simulink model "LQR_sim"  (R2018b)
settings: Solver=ode45  StartTime=0.0  StopTime=tf  RelTol=1e-3  EnableMultiTasking=on
values from neighbouring files (symbols this model uses):
  a = 0.92    [LQR.m]
  b = 0.5    [LQR.m]
  initial = [0,10]    [LQR.m]
  J = 6689.281*10^-6    (= 0.006689281)    [LQR.m]    (also in optimalcontrol.m)
  L = 284.84*10^-3    (= 0.28484)    [LQR.m]    (also in optimalcontrol.m = 0.5*R*u^2)
  PWMs_fixed = [1619,1638]    [LQR.m]
libraries: aerolibconvert2 x2
settings Model: Creator=lorem  LastModifiedBy=davidefontana
settings DataIOCC: LimitDataPoints=on  SaveFormat=Array
settings OptimizationCC: LifeSpan=inf
settings DebuggingCC: SolverPrmCheckMsg=warning  SFUnexpectedBacktrackingDiag=warning  SFNoUnconditionalDefaultTransitionDiag=warning  SFExecutionAtInitializationDiag=none
settings HardwareCC: ProdBitPerPointer=32  ProdBitPerSizeT=32  ProdBitPerPtrDiffT=32  ProdLargestAtomicFloat=None  ProdIntDivRoundTo=Undefined  ProdEndianess=Unspecified  ProdWordSize=32  ProdHWDeviceType=32-bit Generic
settings ModelReferenceCC: PropagateSignalLabelsOutOfModel=off
settings SFSimCC: SimUseLocalCustomCode=off
settings RTWCC: RTWUseLocalCustomCode=off
settings CodeAppCC: StateflowObjectComments=on
settings GRTTargetCC: TargetLangStandard=C89/C90 (ANSI)  GeneratePreprocessorConditionals=Disable all
settings ConfigComp: CovMetricSettings=dw  CovHtmlReporting=on  CovSaveCumulativeToWorkspaceVar=on  CovSaveSingleToWorkspaceVar=on  CovExternalEMLEnable=off  CovSFcnEnable=off

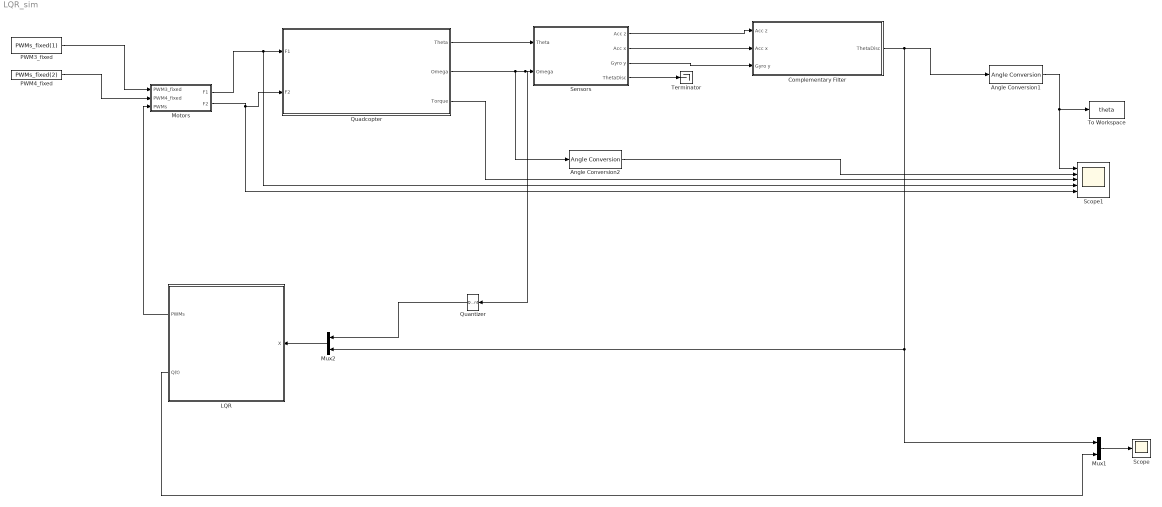
== system LQR_sim ==
  Angle Conversion1 : aerolibconvert2/Angle Conversion  IU=rad  OU=deg
  Angle Conversion2 : aerolibconvert2/Angle Conversion  IU=rad  OU=deg
  Complementary Filter : Subsystem
  LQR : Subsystem
  Motors : Subsystem
  Mux1 : Mux  Inputs=2
  Mux2 : Mux  Inputs=2
  PWM3_fixed : Constant  Value=PWMs_fixed(1)  SampleTime=0.02
  PWM4_fixed : Constant  Value=PWMs_fixed(2)  SampleTime=0.02
  Quadcopter : Subsystem
  Quantizer : Quantizer  QuantizationInterval=0.01  SampleTime=0.02
  Scope : Scope
  Scope1 : Scope  NumInputPorts=5
  Sensors : Subsystem
  Terminator : Terminator
  To Workspace : ToWorkspace  VariableName=theta  SaveFormat=Timeseries  SampleTime=-1
  wires:
  PWM4_fixed/1 -> Motors/2(PWM4_fixed)
  Motors/2(F2) -> Scope1/5, Quadcopter/2(F2)
  Motors/1(F1) -> Scope1/4, Quadcopter/1(F1)
  Sensors/3(Gyro y) -> Complementary Filter/3(Gyro y)
  Sensors/2(Acc x) -> Complementary Filter/2("Acc x ")
  Sensors/1(Acc z) -> Complementary Filter/1(Acc z)
  PWM3_fixed/1 -> Motors/1(PWM3_fixed)
  Angle Conversion1/1 -> Scope1/1, To Workspace/1
  Quadcopter/2(Omega) -> Quantizer/1, Sensors/2(Omega), Angle Conversion2/1
  Quadcopter/1(Theta) -> Sensors/1(Theta)
  Quadcopter/3("Torque ") -> Scope1/3
  Sensors/4(ThetaDisc) -> Terminator/1
  Angle Conversion2/1 -> Scope1/2
  LQR/1(PWMs) -> Motors/3(PWMs)
  Quantizer/1 -> Mux2/1
  Complementary Filter/1(ThetaDisc) -> Mux1/1, Mux2/2, Angle Conversion1/1
  LQR/2(Q(t)) -> Mux1/2
  Mux1/1 -> Scope/1
  Mux2/1 -> LQR/1(X)

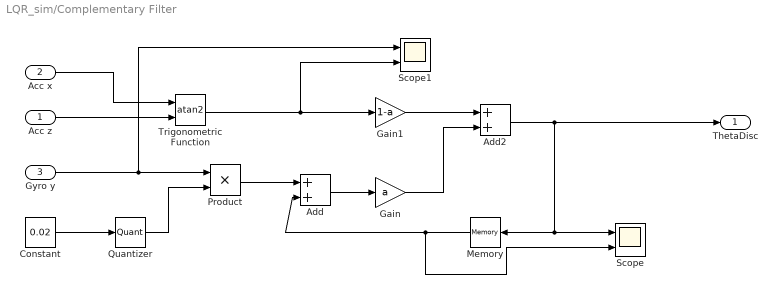
== system LQR_sim/Complementary Filter ==
  Acc z : Inport
  "Acc x " : Inport  Port=2
  Gyro y : Inport  Port=3
  Add : Sum
  Add2 : Sum
  Constant : Constant  Value=0.02
  Gain : Gain  Gain=a
  Gain1 : Gain  Gain=1-a
  Memory : Memory  InitialCondition=deg2rad(initial(2))  InheritSampleTime=on  LinearizeAsDelay=on
  Product : Product
  Quantizer : Quantizer  QuantizationInterval=0.01  SampleTime=0.02
  Scope : Scope  NumInputPorts=2
  Scope1 : Scope  NumInputPorts=2
  Trigonometric Function : Trigonometry  Operator=atan2
  ThetaDisc : Outport
  wires:
  "Acc x "/1 -> Trigonometric Function/1
  Acc z/1 -> Trigonometric Function/2
  Constant/1 -> Quantizer/1
  Gyro y/1 -> Product/1, Scope1/1
  Quantizer/1 -> Product/2
  Product/1 -> Add/1
  Add/1 -> Gain/1
  Gain1/1 -> Add2/1
  Gain/1 -> Add2/2
  Add2/1 -> ThetaDisc/1, Scope/1, Memory/1
  Memory/1 -> Scope/2, Add/2
  Trigonometric Function/1 -> Gain1/1, Scope1/2

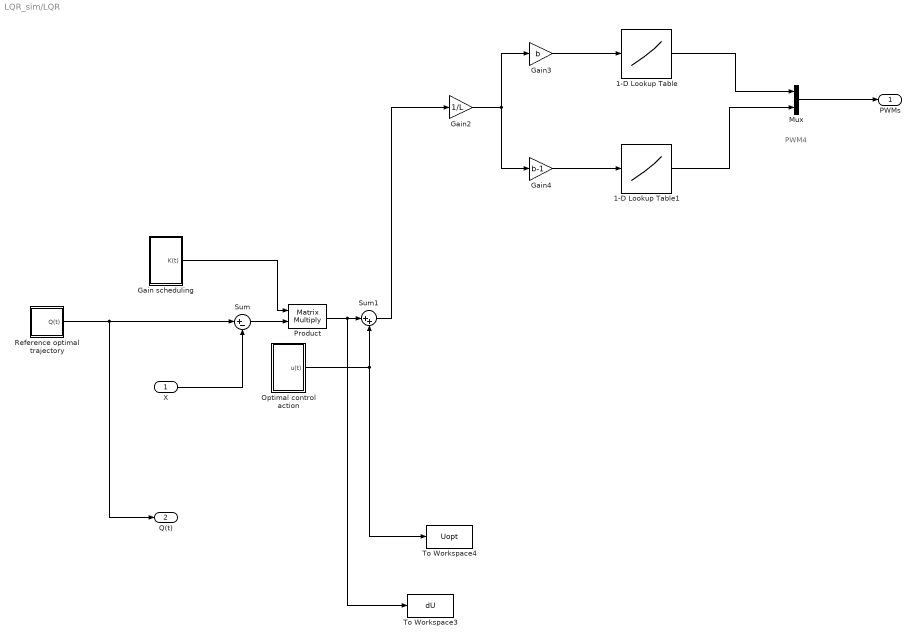
== system LQR_sim/LQR ==
  note: PWM4
  X : Inport
  1-D Lookup Table : Lookup_n-D  NumberOfTableDimensions=1  BreakpointsForDimension1=[-2,2]  Table=[-138,138]  InternalRulePriority=Speed  RndMeth=Simplest  InputSameDT=on
  1-D Lookup Table1 : Lookup_n-D  NumberOfTableDimensions=1  BreakpointsForDimension1=[-2,2]  Table=[-150.8,150.8]  InternalRulePriority=Speed  RndMeth=Simplest  InputSameDT=on
  Gain scheduling : Subsystem
  Gain2 : Gain  Gain=1/L
  Gain3 : Gain  Gain=b
  Gain4 : Gain  Gain=b-1
  Mux : Mux  Inputs=2
  Optimal control action : Subsystem
  Product : Product  Multiplication=Matrix(*)
  Reference optimal trajectory : Subsystem
  Sum : Sum  Inputs=|+-
  Sum1 : Sum  Inputs=|++
  To Workspace3 : ToWorkspace  VariableName=dU  SaveFormat=Timeseries  SampleTime=-1
  To Workspace4 : ToWorkspace  VariableName=Uopt  SaveFormat=Timeseries  SampleTime=-1
  PWMs : Outport
  Q(t) : Outport  Port=2
  wires:
  Gain scheduling/1(K(t)) -> Product/1
  Gain4/1 -> 1-D Lookup Table1/1
  Sum/1 -> Product/2
  Mux/1 -> PWMs/1
  Optimal control action/1(u(t)) -> To Workspace4/1, Sum1/2
  Gain3/1 -> 1-D Lookup Table/1
  Product/1 -> Sum1/1, To Workspace3/1
  Reference optimal trajectory/1(Q(t)) -> Q(t)/1, Sum/1
  Sum1/1 -> Gain2/1
  1-D Lookup Table1/1 -> Mux/2
  1-D Lookup Table/1 -> Mux/1
  Gain2/1 -> Gain3/1, Gain4/1
  X/1 -> Sum/2

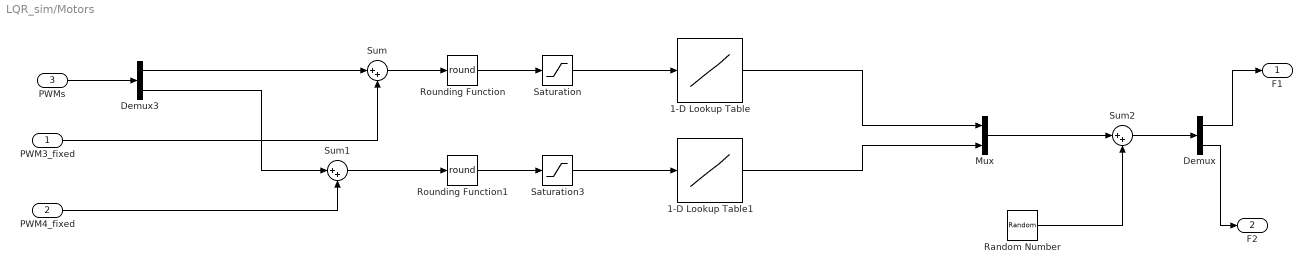
== system LQR_sim/Motors ==
  PWM3_fixed : Inport
  PWM4_fixed : Inport  Port=2
  PWMs : Inport  Port=3
  1-D Lookup Table : Lookup_n-D  NumberOfTableDimensions=1  BreakpointsForDimension1=[1447,1792]  Table=[1,5]  InternalRulePriority=Speed  RndMeth=Simplest  InputSameDT=on
  1-D Lookup Table1 : Lookup_n-D  NumberOfTableDimensions=1  BreakpointsForDimension1=[1455,1832]  Table=[1,5]  InternalRulePriority=Speed  RndMeth=Simplest  InputSameDT=on
  Demux : Demux  Outputs=2
  Demux3 : Demux  Outputs=2
  Mux : Mux  Inputs=2
  Random Number : RandomNumber  Variance=0.036579  SampleTime=0.02
  Rounding Function : Rounding  Operator=round
  Rounding Function1 : Rounding  Operator=round
  Saturation : Saturate  UpperLimit=1792  LowerLimit=1447
  Saturation3 : Saturate  UpperLimit=1832  LowerLimit=1455
  Sum : Sum  Inputs=|++
  Sum1 : Sum  Inputs=|++
  Sum2 : Sum  Inputs=|++
  F1 : Outport
  F2 : Outport  Port=2
  wires:
  PWMs/1 -> Demux3/1
  PWM4_fixed/1 -> Sum1/2
  PWM3_fixed/1 -> Sum/2
  Demux3/1 -> Sum/1
  Demux3/2 -> Sum1/1
  Sum1/1 -> Rounding Function1/1
  Rounding Function1/1 -> Saturation3/1
  Sum/1 -> Rounding Function/1
  Rounding Function/1 -> Saturation/1
  Saturation/1 -> 1-D Lookup Table/1
  Saturation3/1 -> 1-D Lookup Table1/1
  1-D Lookup Table/1 -> Mux/1
  1-D Lookup Table1/1 -> Mux/2
  Mux/1 -> Sum2/1
  Random Number/1 -> Sum2/2
  Sum2/1 -> Demux/1
  Demux/2 -> F2/1
  Demux/1 -> F1/1

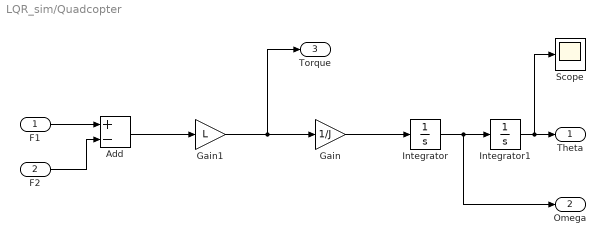
== system LQR_sim/Quadcopter ==
  F1 : Inport
  F2 : Inport  Port=2
  Add : Sum  Inputs=+-
  Gain : Gain  Gain=1/J
  Gain1 : Gain  Gain=L
  Integrator : Integrator  InitialCondition=deg2rad(initial(1))
  Integrator1 : Integrator  InitialCondition=deg2rad(initial(2))
  Scope : Scope
  Theta : Outport
  Omega : Outport  Port=2
  "Torque " : Outport  Port=3
  wires:
  Gain/1 -> Integrator/1
  Integrator/1 -> Omega/1, Integrator1/1
  F2/1 -> Add/2
  F1/1 -> Add/1
  Add/1 -> Gain1/1
  Gain1/1 -> "Torque "/1, Gain/1
  Integrator1/1 -> Scope/1, Theta/1

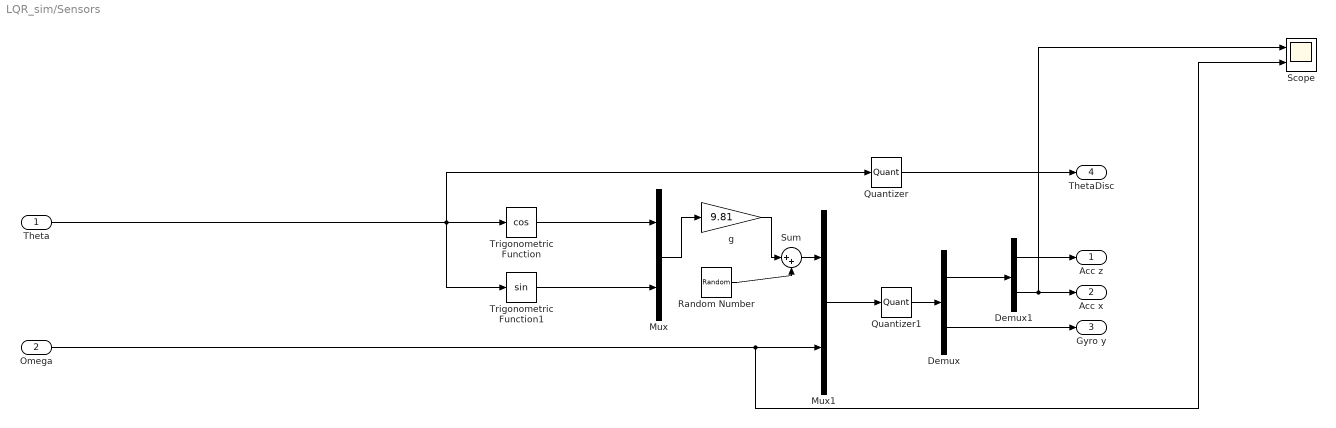
== system LQR_sim/Sensors ==
  Theta : Inport
  Omega : Inport  Port=2
  Demux : Demux  Outputs=2
  Demux1 : Demux  Outputs=2
  Mux : Mux  Inputs=2
  Mux1 : Mux  Inputs=2
  Quantizer : Quantizer  QuantizationInterval=0.01  SampleTime=0.02
  Quantizer1 : Quantizer  QuantizationInterval=0.01  SampleTime=0.02
  Random Number : RandomNumber  Variance=0.0127  SampleTime=0
  Scope : Scope  NumInputPorts=2
  Sum : Sum  Inputs=|++
  Trigonometric Function : Trigonometry  Operator=cos
  Trigonometric Function1 : Trigonometry
  g : Gain  Gain=9.81
  Acc z : Outport
  Acc x : Outport  Port=2
  Gyro y : Outport  Port=3
  ThetaDisc : Outport  Port=4
  wires:
  Trigonometric Function1/1 -> Mux/2
  Trigonometric Function/1 -> Mux/1
  Mux/1 -> g/1
  Mux1/1 -> Quantizer1/1
  Quantizer1/1 -> Demux/1
  Demux/2 -> Gyro y/1
  Demux/1 -> Demux1/1
  Demux1/1 -> Acc z/1
  Omega/1 -> Scope/2, Mux1/2
  Theta/1 -> Quantizer/1, Trigonometric Function1/1, Trigonometric Function/1
  Demux1/2 -> Scope/1, Acc x/1
  Quantizer/1 -> ThetaDisc/1
  g/1 -> Sum/1
  Random Number/1 -> Sum/2
  Sum/1 -> Mux1/1

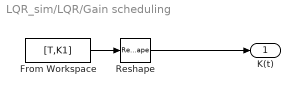
== system LQR_sim/LQR/Gain scheduling ==
  From Workspace : FromWorkspace  VariableName=[T,K1]  SampleTime=0
  Reshape : Reshape  OutputDimensionality=Row vector (2-D)
  K(t) : Outport
  wires:
  From Workspace/1 -> Reshape/1
  Reshape/1 -> K(t)/1

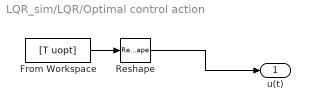
== system LQR_sim/LQR/Optimal control action ==
  From Workspace : FromWorkspace  VariableName=[T uopt]  SampleTime=0
  Reshape : Reshape  OutputDimensionality=Column vector (2-D)
  u(t) : Outport
  wires:
  Reshape/1 -> u(t)/1
  From Workspace/1 -> Reshape/1

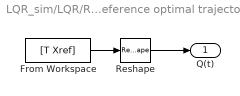
== system LQR_sim/LQR/Reference optimal trajectory ==
  From Workspace : FromWorkspace  VariableName=[T Xref]  SampleTime=0
  Reshape : Reshape  OutputDimensionality=Column vector (2-D)
  Q(t) : Outport
  wires:
  From Workspace/1 -> Reshape/1
  Reshape/1 -> Q(t)/1
